simulink model "p5p3b_"  (Simulink 9.2)
settings: Solver=ode45  StartTime=0.0  StopTime=500  RelTol=1e-3  EnableMultiTasking=on
undefined symbols (not defined in the file or in its folder): Kpd, Td, Tf
libraries: simulink x2
settings Model: Creator=markh  LastModifiedBy=Flemmen
settings DataIOCC: SignalLoggingName=sigsOut
settings OptimizationCC: InitFltsAndDblsToZero=on
settings DebuggingCC: SaveWithParameterizedLinksMsg=none  SignalResolutionControl=TryResolveAllWithWarning  MultiTaskDSMMsg=warning  MultiTaskCondExecSysMsg=none
settings HardwareCC: TargetUnknown=on
settings GRTTargetCC: TargetFcnLib=ansi_tfl_tmw.mat

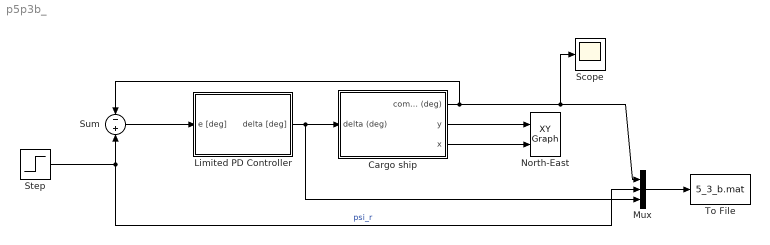
== system p5p3b_ ==
  Cargo ship : Subsystem  mask(Simple shipmodel for a cargo ship){noise=on, current=off, logic=off}
      mask prompts: noise "measurement noise"; logic "waves"
      mask help:
      | Measurement noise:
      | 	checked = noise on
      | 	unchecked = noise off
      |
      | Current:
      | 	checked = current on
      | 	unchecked = current off
      |
      | Waves:
      | 	checked = waves on
      | 	unchecked = waves off
      |
      | Author: Jørgen Spjøtvold, 9/10-2003
      | TTK 4115 Linear system theory.
      | Modified by Jostein Bakkeheim 26/10-2006
  Limited PD Controller : Subsystem
  Mux : Mux  Inputs=3
  North-East : simulink/Sinks/XY Graph  xmin=-5000  xmax=5000  ymin=-5000  ymax=5000  st=-1
  Scope : Scope
  Step : Step  After=35  SampleTime=0
  Sum : Sum  Inputs=-|+
  To File : ToFile  Filename=5_3_b.mat
  wires:
  Cargo ship/3(x) -> North-East/2
  Cargo ship/2(y) -> North-East/1
  Step/1 -> Mux/2, Sum/2  "psi_r"
  Cargo ship/1(compass (deg)) -> Mux/1, Scope/1, Sum/1
  Sum/1 -> Limited PD Controller/1(e [deg])
  Mux/1 -> To File/1
  Limited PD Controller/1(delta [deg]) -> Mux/3, Cargo ship/1(delta (deg))

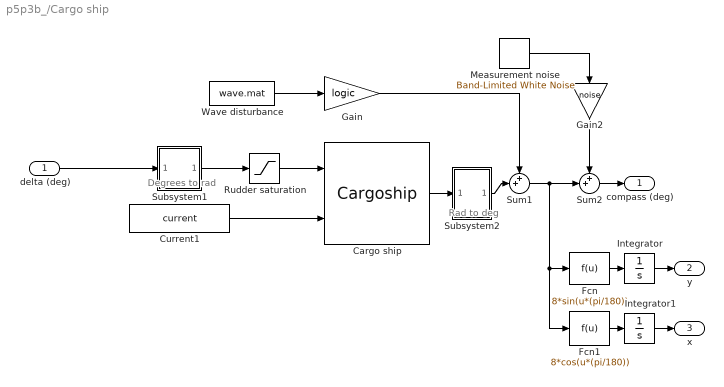
== system p5p3b_/Cargo ship ==
  note: Degrees to rad
  note: Rad to deg
  delta (deg) : Inport
  Cargo ship : S-Function  FunctionName=Cargoship  SFunctionDeploymentMode=off  EnableBusSupport=off  mask(Cargo ship){}
      mask help:
      | S-function which simulates a cargo ship.
      |
      | Author: Jørgen Spjøtvold
      | 20.10-2003
      | Modified by Jostein Bakkeheim 27.10.2006
  Current1 : Constant  Value=current
  Fcn : Fcn  Expr=8*sin(u*(pi/180))
  Fcn1 : Fcn  Expr=8*cos(u*(pi/180))
  Gain : Gain  Gain=logic  SaturateOnIntegerOverflow=on  OutDataTypeStr=Inherit: Same as input  ParamDataTypeStr=Inherit: Same as input
  Gain2 : Gain  Gain=noise  SaturateOnIntegerOverflow=on  OutDataTypeStr=Inherit: Same as input  ParamDataTypeStr=Inherit: Same as input
  Integrator : Integrator
  Integrator1 : Integrator
  Measurement noise : simulink/Sources/Band-Limited White Noise  Cov=[0.001]  Ts=.5  seed=[23341]
  Rudder saturation : Saturate  UpperLimit=45*(pi/180)  LowerLimit=-45*(pi/180)
  Subsystem1 : Subsystem  mask(degrees to radians){}
      mask help: Converts degrees to radians
      mask Display: fprintf('D2R');
  Subsystem2 : Subsystem  mask(radians to degrees){}
      mask help: Converts radians to degrees
      mask Display: fprintf('R2D');
  Sum1 : Sum  Inputs=++|  SaturateOnIntegerOverflow=on
  Sum2 : Sum  Inputs=++|  SaturateOnIntegerOverflow=on
  Wave disturbance : FromFile  FileName=wave.mat  SampleTime=0
  compass (deg) : Outport
  y : Outport  Port=2
  x : Outport  Port=3
  wires:
  delta (deg)/1 -> Subsystem1/1(In1)
  Fcn/1 -> Integrator/1
  Integrator/1 -> y/1
  Fcn1/1 -> Integrator1/1
  Integrator1/1 -> x/1
  Wave disturbance/1 -> Gain/1
  Subsystem2/1(Out1) -> Sum1/2
  Gain/1 -> Sum1/1
  Sum1/1 -> Fcn/1, Fcn1/1, Sum2/2
  Cargo ship/1 -> Subsystem2/1(In1)
  Subsystem1/1(Out1) -> Rudder saturation/1
  Rudder saturation/1 -> Cargo ship/1
  Sum2/1 -> compass (deg)/1
  Measurement noise/1 -> Gain2/1
  Gain2/1 -> Sum2/1
  Current1/1 -> Cargo ship/2

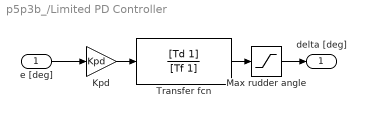
== system p5p3b_/Limited PD Controller ==
  e [deg] : Inport
  Kpd : Gain  Gain=Kpd
  Max rudder angle : Saturate  UpperLimit=45  LowerLimit=-45
  Transfer fcn : TransferFcn  Numerator=[Td 1]  Denominator=[Tf 1]
  delta [deg] : Outport
  wires:
  Kpd/1 -> Transfer fcn/1
  e [deg]/1 -> Kpd/1
  Max rudder angle/1 -> delta [deg]/1
  Transfer fcn/1 -> Max rudder angle/1

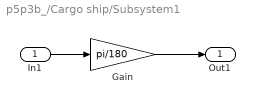
== system p5p3b_/Cargo ship/Subsystem1 ==
  In1 : Inport
  Gain : Gain  Gain=pi/180  SaturateOnIntegerOverflow=on  OutDataTypeStr=Inherit: Same as input  ParamDataTypeStr=Inherit: Same as input
  Out1 : Outport
  wires:
  Gain/1 -> Out1/1
  In1/1 -> Gain/1

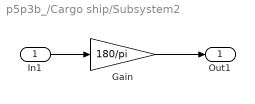
== system p5p3b_/Cargo ship/Subsystem2 ==
  In1 : Inport
  Gain : Gain  Gain=180/pi  SaturateOnIntegerOverflow=on  OutDataTypeStr=Inherit: Same as input  ParamDataTypeStr=Inherit: Same as input
  Out1 : Outport
  wires:
  Gain/1 -> Out1/1
  In1/1 -> Gain/1
